simulink model "planta"  (R2023a)
settings: Solver=VariableStepAuto  StartTime=0.0  StopTime=1000  RelTol=1e-3
settings Model: Creator=empg0  LastModifiedBy=empg0

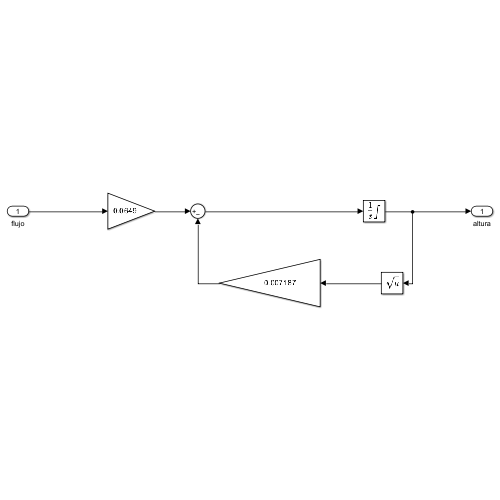
[thumbnail: Simulink's stored preview of the top-level diagram]
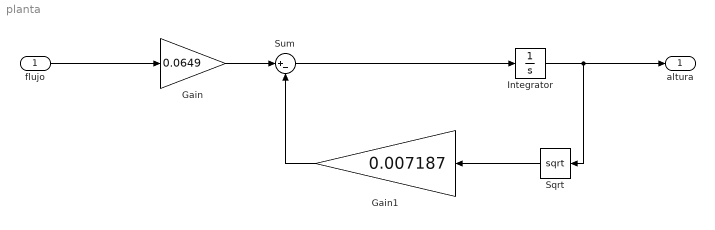
== system planta ==
  flujo : Inport
  Gain : Gain  Gain=0.0649
  Gain1 : Gain  Gain=0.007187
  Integrator : Integrator  LimitOutput=on  UpperSaturationLimit=0.62  LowerSaturationLimit=0
  Sqrt : Sqrt
  Sum : Sum  Inputs=|+-
  altura : Outport
  wires:
  Integrator/1 -> altura/1, Sqrt/1
  flujo/1 -> Gain/1
  Sum/1 -> Integrator/1
  Sqrt/1 -> Gain1/1
  Gain1/1 -> Sum/2
  Gain/1 -> Sum/1
